simulink model "MassSpringDamper_nonlinear"  (R2019a)
settings: Solver=VariableStepAuto  StartTime=0.0  StopTime=T_sim  RelTol=1e-3
values from neighbouring files (symbols this model uses):
  A = [ 0       1 ... (first row only)    [MassSpringDamper_nonlinear_init.m]
  A_nl = [0 ... (first row only)    [MassSpringDamper_nonlinear_init.m]
  B = [ 0 ... (first row only)    [MassSpringDamper_nonlinear_init.m]
  C = [1  0]    [MassSpringDamper_nonlinear_init.m]
  D = [0]    [MassSpringDamper_nonlinear_init.m]
  T_s = 1/fs    (= 0.005)    [MassSpringDamper_nonlinear_init.m]
settings Model: Creator=alexander  LastModifiedBy=alexander

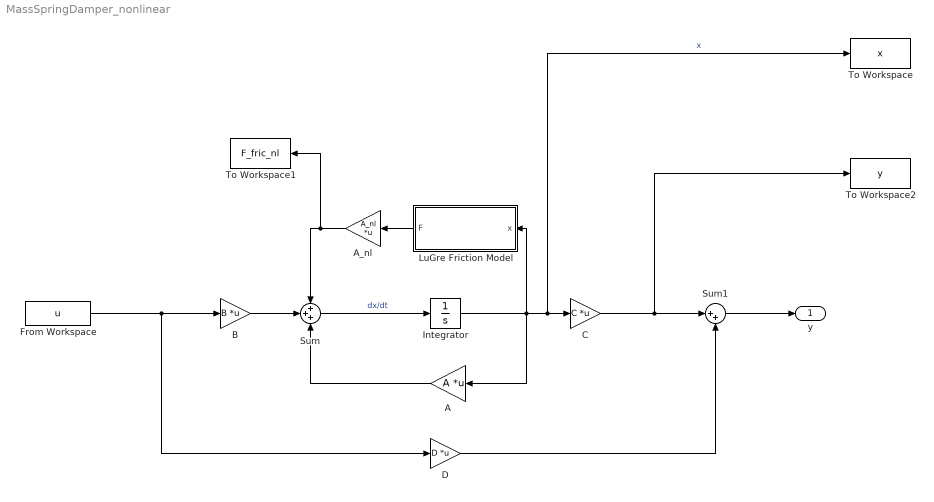
== system MassSpringDamper_nonlinear ==
  A : Gain  Gain=A  Multiplication=Matrix(K*u)
  A_nl : Gain  Gain=A_nl  Multiplication=Matrix(K*u)
  B : Gain  Gain=B  Multiplication=Matrix(K*u)
  C : Gain  Gain=C  Multiplication=Matrix(K*u)
  D : Gain  Gain=D  Multiplication=Matrix(K*u)
  From Workspace : FromWorkspace  VariableName=u  SampleTime=T_s
  Integrator : Integrator
  LuGre Friction Model : Subsystem
  Sum : Sum  Inputs=+++
  Sum1 : Sum  Inputs=|++
  To Workspace : ToWorkspace  VariableName=x  SampleTime=T_s
  To Workspace1 : ToWorkspace  VariableName=F_fric_nl  SampleTime=T_s
  To Workspace2 : ToWorkspace  VariableName=y  SampleTime=T_s
  y : Outport
  wires:
  From Workspace/1 -> D/1, B/1
  Sum/1 -> Integrator/1  "dx/dt"
  Integrator/1 -> LuGre Friction Model/1(x), A/1, To Workspace/1, C/1  "x"
  C/1 -> To Workspace2/1, Sum1/1
  Sum1/1 -> y/1
  D/1 -> Sum1/2
  A_nl/1 -> To Workspace1/1, Sum/1
  A/1 -> Sum/3
  B/1 -> Sum/2
  LuGre Friction Model/1(F) -> A_nl/1

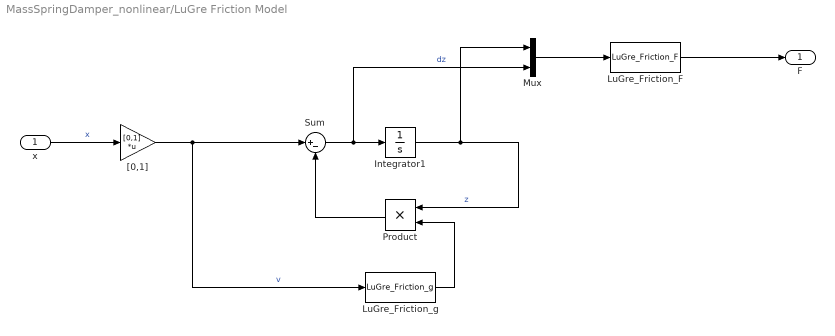
== system MassSpringDamper_nonlinear/LuGre Friction Model ==
  x : Inport
  Integrator1 : Integrator
  LuGre_Friction_F : MATLABFcn  MATLABFcn=LuGre_Friction_F
  LuGre_Friction_g : MATLABFcn  MATLABFcn=LuGre_Friction_g
  Mux : Mux  Inputs=2
  Product : Product
  Sum : Sum  Inputs=|+-
  "[0,1]" : Gain  Gain=[0,1]  Multiplication=Matrix(K*u)
  F : Outport
  wires:
  Integrator1/1 -> Mux/1, Product/1  "z"
  Sum/1 -> Mux/2, Integrator1/1  "dz"
  Product/1 -> Sum/2
  LuGre_Friction_g/1 -> Product/2
  x/1 -> "[0,1]"/1  "x"
  Mux/1 -> LuGre_Friction_F/1
  LuGre_Friction_F/1 -> F/1
  "[0,1]"/1 -> LuGre_Friction_g/1, Sum/1  "v"
